simulink model "Simple_Pendulum_Motion"  (R2023a)
settings: Solver=ode45  StartTime=0.0  StopTime=10.0  MaxStep=1e-3  RelTol=1e-3
undefined symbols (not defined in the file): g, L
settings Model: Creator=EMRIX  LastModifiedBy=EMRIX

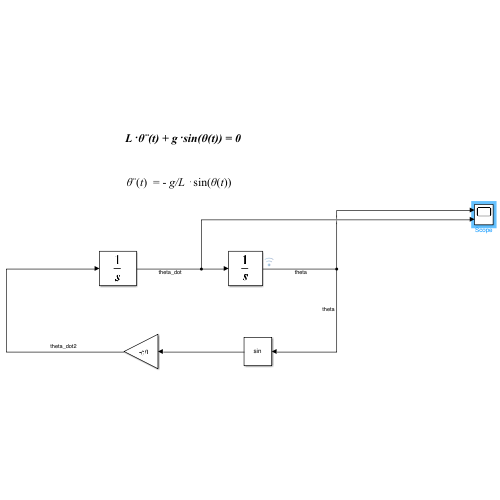
[thumbnail: Simulink's stored preview of the top-level diagram]
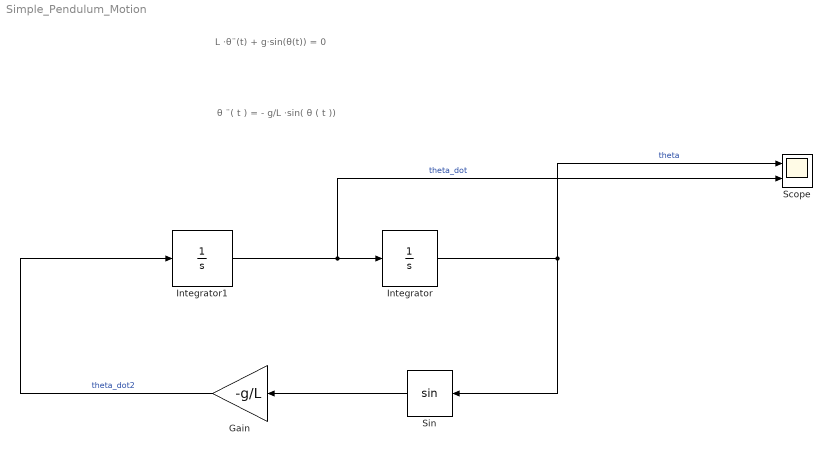
== system Simple_Pendulum_Motion ==
  note: θ ¨( t ) = - g/L ⋅sin( θ ( t ))
  note: L ⋅θ¨(t) + g⋅sin(θ(t)) = 0
  Gain : Gain  Gain=-g/L
  Integrator : Integrator  InitialCondition=2
  Integrator1 : Integrator
  Scope : Scope  NumInputPorts=2
  Sin : Trigonometry
  wires:
  Integrator1/1 -> Scope/2, Integrator/1  "theta_dot"
  Integrator/1 -> Scope/1, Sin/1  "theta"
  Sin/1 -> Gain/1
  Gain/1 -> Integrator1/1  "theta_dot2"
